simulink model "pid_ex1"  (R2018b)
settings: Solver=ode45  StartTime=0.0  StopTime=10.0  RelTol=1e-3  EnableMultiTasking=on
PreLoadFcn:
  | Ts = 0.2;
settings Model: Creator=nicholas  LastModifiedBy=Alexander
settings DataIOCC: LimitDataPoints=on  SaveFormat=Array  SignalLoggingName=sigsOut
settings OptimizationCC: ExpressionDepthLimit=2147483647  InitFltsAndDblsToZero=on  LifeSpan=inf
settings DebuggingCC: SaveWithParameterizedLinksMsg=none  UnderspecifiedInitializationDetection=Classic  MergeDetectMultiDrivingBlocksExec=none  SignalResolutionControl=TryResolveAllWithWarning  MultiTaskDSMMsg=warning  MultiTaskCondExecSysMsg=none  ParameterPrecisionLossMsg=none  FcnCallInpInsideContextMsg=warning  AllowSymbolicDim=off  StateNameClashWarn=warning  LibraryContextMissingDiagnostic=none  SFUnexpectedBacktrackingDiag=warning  SFNoUnconditionalDefaultTransitionDiag=warning  SFExecutionAtInitializationDiag=none
settings HardwareCC: ProdBitPerPointer=32  ProdBitPerSizeT=32  ProdBitPerPtrDiffT=32  ProdLargestAtomicFloat=None  ProdIntDivRoundTo=Undefined  ProdEndianess=Unspecified  ProdWordSize=32  ProdHWDeviceType=32-bit Generic  TargetUnknown=on
settings ModelReferenceCC: PropagateSignalLabelsOutOfModel=off
settings SFSimCC: SimUseLocalCustomCode=off
settings RTWCC: RTWUseLocalCustomCode=off
settings CodeAppCC: StateflowObjectComments=on
settings GRTTargetCC: TargetFcnLib=ansi_tfl_tmw.mat  TargetLangStandard=C89/C90 (ANSI)  GeneratePreprocessorConditionals=Disable all  CombineOutputUpdateFcns=off  GRTInterface=on
settings ConfigComp: CovMetricSettings=dw  CovHtmlReporting=on  CovSaveCumulativeToWorkspaceVar=on  CovSaveSingleToWorkspaceVar=on  CovExternalEMLEnable=off  CovSFcnEnable=off

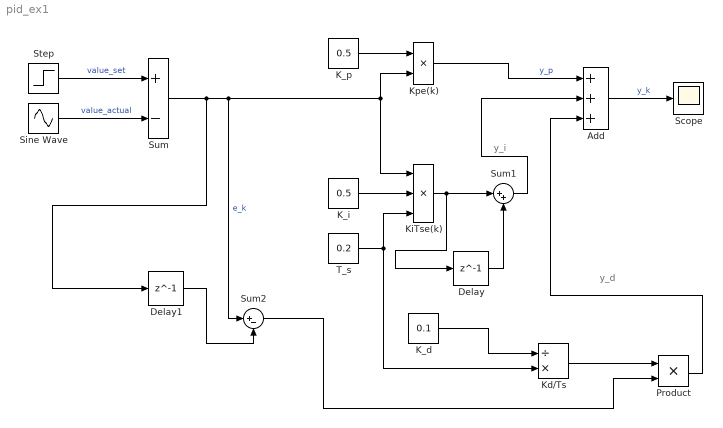
== system pid_ex1 ==
  note: y_i
  note: y_d
  Add : Sum  Inputs=+++
  Delay : Delay  DelayLength=1
  Delay1 : Delay  DelayLength=1
  K_d : Constant  Value=0.1
  K_i : Constant  Value=0.5
  K_p : Constant  Value=0.5
  Kd/Ts : Product  Inputs=/*
  KiTse(k) : Product  Inputs=3
  Kpe(k) : Product
  Product : Product
  Scope : Scope
  Sine Wave : Sin  SampleTime=Ts
  Step : Step  SampleTime=Ts
  Sum : Sum  Inputs=+-  SaturateOnIntegerOverflow=on  InputSameDT=on  OutDataTypeStr=Inherit: Same as first input
  Sum1 : Sum  Inputs=|++
  Sum2 : Sum  Inputs=|+-
  T_s : Constant  Value=0.2
  wires:
  Add/1 -> Scope/1  "y_k"
  Step/1 -> Sum/1  "value_set"
  Sine Wave/1 -> Sum/2  "value_actual"
  Sum/1 -> Delay1/1, KiTse(k)/1, Kpe(k)/2, Sum2/1  "e_k"
  K_p/1 -> Kpe(k)/1
  Kpe(k)/1 -> Add/1  "y_p"
  KiTse(k)/1 -> Delay/1, Sum1/1
  Sum1/1 -> Add/2
  K_i/1 -> KiTse(k)/2
  T_s/1 -> Kd/Ts/2, KiTse(k)/3
  Delay/1 -> Sum1/2
  K_d/1 -> Kd/Ts/1
  Kd/Ts/1 -> Product/1
  Delay1/1 -> Sum2/2
  Sum2/1 -> Product/2
  Product/1 -> Add/3
